simulink model "roll_ap_testharness"  (R2013a)
settings: Solver=FixedStepDiscrete  StartTime=0.0  StopTime=25  FixedStep=1/40  RelTol=1e-3
undefined symbols (not defined in the file): dispGain, hdgGain, intGain, rateGain, sigbuilder_block
libraries: simulink x1
settings Model: CovMetricSettings=dcmrw  CovHTMLOptions=-sRT=1 -aTS=1 -bRG=1 -bTC=1 -hTR=0 -nFC=0 -scm=1 -bcm=1 -xEv=0  CovModelRefEnable=all  Creator=syoon  LastModifiedBy=syoon
settings OptimizationCC: BlockReduction=off  InlineParams=on  InlineInvariantSignals=on  EfficientFloat2IntCast=on  EfficientMapNaN2IntZero=off  OptimizeModelRefInitCode=on  MaxStackSize=inf
settings DebuggingCC: SignalInfNanChecking=error  ReadBeforeWriteMsg=EnableAllAsError  WriteAfterWriteMsg=EnableAllAsError  WriteAfterReadMsg=EnableAllAsError  AlgebraicLoopMsg=error  ArtificialAlgebraicLoopMsg=error  SaveWithDisabledLinksMsg=error  SaveWithParameterizedLinksMsg=error  UnderspecifiedInitializationDetection=Simplified  BlockPriorityViolationMsg=error  MaxConsecutiveZCsMsg=warning  SolverPrmCheckMsg=error  InheritedTsInSrcMsg=error  DiscreteInheritContinuousMsg=error  SingleTaskRateTransMsg=error  TasksWithSamePriorityMsg=error  SigSpecEnsureSampleTimeMsg=error  IntegerOverflowMsg=error  ParameterUnderflowMsg=error  ParameterPrecisionLossMsg=error  ParameterTunabilityLossMsg=error  UnnecessaryDatatypeConvMsg=warning  VectorMatrixConversionMsg=error  SignalLabelMismatchMsg=error  UnconnectedInputMsg=error  UnconnectedOutputMsg=error  UnconnectedLineMsg=error  UniqueDataStoreMsg=error  BusObjectLabelMismatch=error  RootOutportRequireBusObject=error  ModelReferenceIOMsg=error  ModelReferenceIOMismatchMessage=error  ModelReferenceCSMismatchMessage=warning  UnknownTsInhSupMsg=error  ModelReferenceDataLoggingMessage=error  ModelReferenceExtraNoncontSigs=none  StrictBusMsg=ErrorOnBusTreatedAsVector  NonBusSignalsTreatedAsBus=error
settings HardwareCC: ProdHWDeviceType=Generic->32-bit Embedded Processor
settings RTWCC: SystemTargetFile=ert.tlc  TemplateMakefile=ert_default_tmf  Description=Embedded Coder  GenerateReport=on  ProcessScript=ert_make_rtw_hook  IncludeHyperlinkInReport=on  LaunchReport=on  GenerateTraceInfo=on  GenerateTraceReport=on  GenerateTraceReportSl=on  GenerateTraceReportSf=on  GenerateTraceReportEml=on  GenerateCodeMetricsReport=on
settings CodeAppCC: IgnoreCustomStorageClasses=off
settings ERTTargetCC: InlinedParameterPlacement=Hierarchical  ERTCustomFileTemplate=example_file_process.tlc

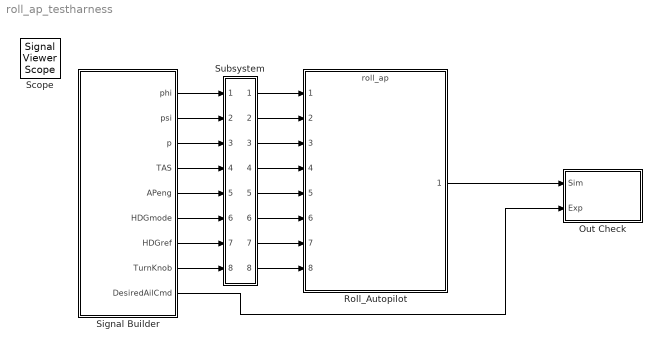
== system roll_ap_testharness ==
  Out Check : Subsystem
  Roll_Autopilot : ModelReference  ModelNameDialog=roll_ap  ParameterArgumentNames=dispGain,intGain,rateGain,hdgGain  ParameterArgumentValues=1.0, 1.0, 3.0, 0.015  SimulationMode=Normal  ModelReferenceVersion=1.164  CopyOfModelName=roll_ap  DefaultDataLogging=on
  Signal Builder : Subsystem  Tag=STV Subsys  LoadFcn=sigbuilder_block('load',[112.5 42 519.75 399.75 ]);  StartFcn=sigbuilder_block('start');  StopFcn=sigbuilder_block('stop');  ClipboardFcn=sigbuilder_block('clipboard');  mask(Sigbuilder block){}
      mask init:
      | if ~strcmp(get_param(bdroot(gcb),'SimulationStatus'),'stopped'),tuvar = sigbuilder_block('maskInit'); end
      settings: CopyFcn=sigbuilder_block('copy');  DeleteFcn=sigbuilder_block('delete');  ModelCloseFcn=sigbuilder_block('modelClose');  PreSaveFcn=sigbuilder_block('preSave');  PauseFcn=sigbuilder_block('pause');  ContinueFcn=sigbuilder_block('continue');  NameChangeFcn=sigbuilder_block('namechange');  OpenFcn=sigbuilder_block('open',[49.5 50.25 519.75 399.75 ]);  CloseFcn=sigbuilder_block('close');
      mask Display: plot(0, 0, 100, 100,[2, 2, 32, 32, 2], [68, 8, 8, 68, 68],[32, 2], [38, 38], [32, 19, 2],[53, 60, 44], [32, 17, 17, 2],[16, 16, 31, 31]);txt = getActiveGroup(gcbh);text(2, 100, txt,'verticalAlignment', 'top');
  Subsystem : Subsystem
      mask Display: disp('Cast')
  Scope : SignalViewerScope  IOType=viewer  NumInputPorts=3  RefreshTime=0.035000
      settings: TimeRange=25  YMin=-20~-20~-1  YMax=10~10~1
  wires:
  Roll_Autopilot/1 -> Out Check/1(Sim)
  Signal Builder/9(DesiredAilCmd) -> Out Check/2(Exp)
  Signal Builder/4(TAS) -> Subsystem/4(In4)
  Signal Builder/2(psi) -> Subsystem/2(In2)
  Signal Builder/1(phi) -> Subsystem/1(In1)
  Signal Builder/3(p) -> Subsystem/3(In3)
  Signal Builder/5(APeng) -> Subsystem/5(In5)
  Signal Builder/8(TurnKnob) -> Subsystem/8(In8)
  Signal Builder/7(HDGref) -> Subsystem/7(In7)
  Signal Builder/6(HDGmode) -> Subsystem/6(In6)
  Subsystem/1(Out1) -> Roll_Autopilot/1
  Subsystem/2(Out2) -> Roll_Autopilot/2
  Subsystem/3(Out3) -> Roll_Autopilot/3
  Subsystem/6(Out6) -> Roll_Autopilot/6
  Subsystem/5(Out5) -> Roll_Autopilot/5
  Subsystem/4(Out4) -> Roll_Autopilot/4
  Subsystem/7(Out7) -> Roll_Autopilot/7
  Subsystem/8(Out8) -> Roll_Autopilot/8

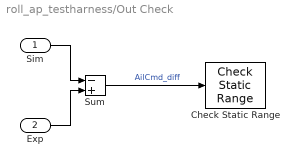
== system roll_ap_testharness/Out Check ==
  Sim : Inport
  Exp : Inport  Port=2
  Check Static Range : simulink/Model Verification/Check  Static Range  Description=-0.1 <= u <= 0.1  max=0.1  max_included=on  min=-0.1  min_included=on  enabled=on  stopWhenAssertionFail=on  export=off  icon=graphic
  Sum : Sum  Inputs=-+
  wires:
  Sim/1 -> Sum/1
  Exp/1 -> Sum/2
  Sum/1 -> Check Static Range/1  "AilCmd_diff"

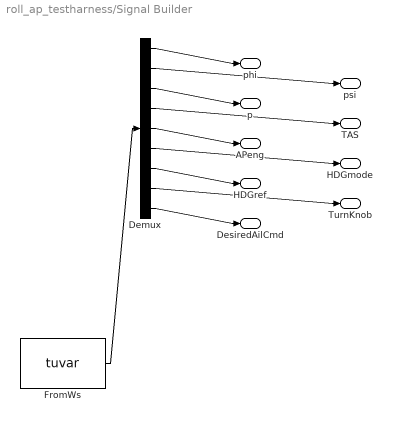
== system roll_ap_testharness/Signal Builder ==
  Demux : Demux  Tag=STV Demux  Outputs=9
  FromWs : FromWorkspace  Tag=STV FromWs  VariableName=tuvar  SampleTime=0
  phi : Outport  Tag=STV Outport
  psi : Outport  Tag=STV Outport  Port=2
  p : Outport  Tag=STV Outport  Port=3
  TAS : Outport  Tag=STV Outport  Port=4
  APeng : Outport  Tag=STV Outport  Port=5
  HDGmode : Outport  Tag=STV Outport  Port=6
  HDGref : Outport  Tag=STV Outport  Port=7
  TurnKnob : Outport  Tag=STV Outport  Port=8
  DesiredAilCmd : Outport  Tag=STV Outport  Port=9
  wires:
  FromWs/1 -> Demux/1
  Demux/1 -> phi/1
  Demux/2 -> psi/1
  Demux/3 -> p/1
  Demux/4 -> TAS/1
  Demux/5 -> APeng/1
  Demux/6 -> HDGmode/1
  Demux/7 -> HDGref/1
  Demux/8 -> TurnKnob/1
  Demux/9 -> DesiredAilCmd/1

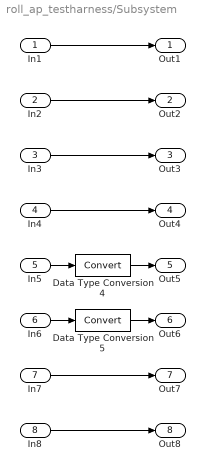
== system roll_ap_testharness/Subsystem ==
  In1 : Inport
  In2 : Inport  Port=2
  In3 : Inport  Port=3
  In4 : Inport  Port=4
  In5 : Inport  Port=5
  In6 : Inport  Port=6
  In7 : Inport  Port=7
  In8 : Inport  Port=8
  Data Type Conversion4 : DataTypeConversion
  Data Type Conversion5 : DataTypeConversion
  Out1 : Outport
  Out2 : Outport  Port=2
  Out3 : Outport  Port=3
  Out4 : Outport  Port=4
  Out5 : Outport  Port=5
  Out6 : Outport  Port=6
  Out7 : Outport  Port=7
  Out8 : Outport  Port=8
  wires:
  In3/1 -> Out3/1
  In2/1 -> Out2/1
  In1/1 -> Out1/1
  Data Type Conversion5/1 -> Out6/1
  In6/1 -> Data Type Conversion5/1
  Data Type Conversion4/1 -> Out5/1
  In5/1 -> Data Type Conversion4/1
  In4/1 -> Out4/1
  In8/1 -> Out8/1
  In7/1 -> Out7/1
